simulink model "dragrace"  (R2021a)
settings: Solver=FixedStepAuto  StartTime=0.0  StopTime=t_final  FixedStep=t_step  RelTol=1e-3
values from neighbouring files (symbols this model uses):
  c_R = 0.015    [data_analysis.m]
  F_Reib = 0    [data_analysis.m]
  gamma = 0    [data_analysis.m]
  lambda = 1    [data_analysis.m]
  m = 2000    [data_analysis.m]
  M_Brems = 0    [data_analysis.m]
  MaxBremsmoment = 1000    [data_analysis.m]
  r = 33.55    [data_analysis.m]
  S_0 = 0    [data_analysis.m]
  v_0 = 0    [data_analysis.m]
  v_L = 0    [data_analysis.m]
settings Model: Creator=62958  LastModifiedBy=62958
settings SolverCC: AlgebraicLoopSolver=TrustRegion
settings DebuggingCC: SFMachineParentedDataDiag=warning
settings HardwareCC: ProdHWDeviceType=AMD->x86-64 (Windows64)

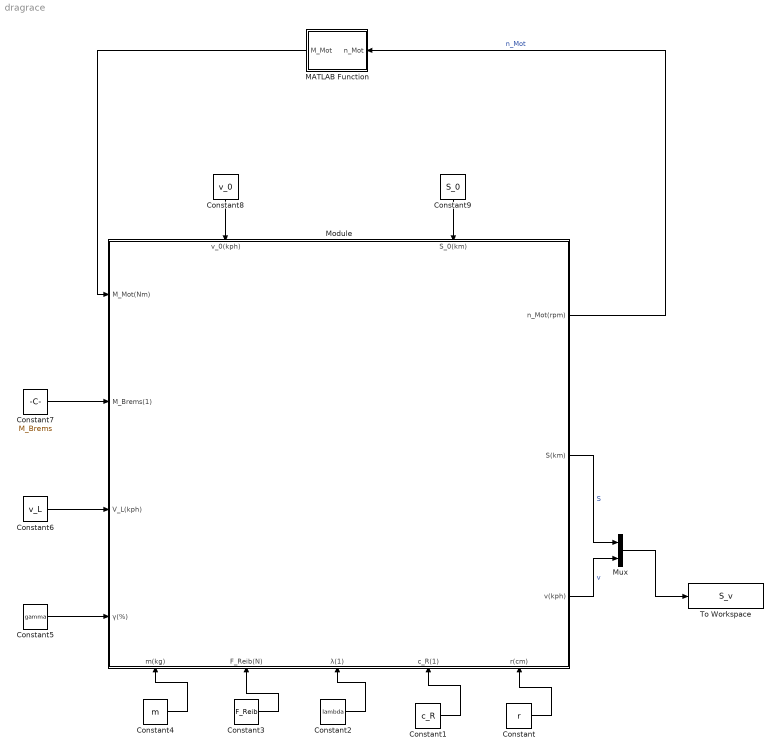
== system dragrace ==
  Constant : Constant  Value=r
  Constant1 : Constant  Value=c_R
  Constant2 : Constant  Value=lambda
  Constant3 : Constant  Value=F_Reib
  Constant4 : Constant  Value=m
  Constant5 : Constant  Value=gamma
  Constant6 : Constant  Value=v_L
  Constant7 : Constant  Value=M_Brems
  Constant8 : Constant  Value=v_0
  Constant9 : Constant  Value=S_0
  MATLAB Function : MATLAB Function  TreatAsAtomicUnit=on
  Module : Subsystem
      settings: PortSchema="{\"entries\":[{\"content\":{\"sides\":[{\"content\":{\"connectorIds\":[\"In1\",\"In2\",\"In3\",\"In4\"]},\"type\":\"ConnectorPlacement.EquallySpacedRectSide\",\"uuid\":\"ac678796-a959-4d6d-9319-846a0b7c832f\"},{\"content\":{\"connectorIds\":[\"Out1\",\"Out2\",\"Out3\"],\"side\":\"RIGHT\"},\"type\":\"ConnectorPlacement.EquallySpacedRectSide\",\"uuid\":\"19604558-b17b-4c8e-bdf8-e9ba0ab768c7\"},{\"content\":{\"connectorIds\":[\"In5\",\"In6\"],\"side\":\"TOP\"},\"type\":\"ConnectorPlacement.EquallySpacedRectSide\",\"uuid\":\"2ba52809-0b07-473f-b1d8-e379260c6f0c\"},{\"content\":{\"connectorIds\":[\"In7\",\"In8\",\"In9\",\"In10\",\"In11\"],\"side\":\"BOTTOM\"},\"type\":\"ConnectorPlacement.EquallySpacedRectSide\",\"uuid\":\"6dc63aca-051a-4fee-a312-85b6adf31509\"},{\"content\":{\"connectorIds\":[],\"side\":\"HIDDEN\"},\"type\":\"ConnectorPlacement.EquallySpacedRectSide\",\"uuid\":\"c73a095b-eeaa-49e3-925b-3fbd9f66e33c\"}]},\"type\":\"ConnectorPlacement.EquallySpacedConnector\",\"uuid\":\"c7629ab1-f4a5-46db-a10e-d6706fe7350a\"}],\"packageUris\":[\"http://schema.mathworks.com/mf0/Connector/R2020b\"],\"version\":\"1.0\"}"
  Mux : Mux  Inputs=2
  To Workspace : ToWorkspace  VariableName=S_v  SaveFormat=Timeseries  SampleTime=-1
  wires:
  MATLAB Function/1(M_Mot) -> Module/1(M_Mot(Nm))
  Module/1(n_Mot(rpm)) -> MATLAB Function/1(n_Mot)  "n_Mot"
  Module/3(v(kph)) -> Mux/2  "v"
  Constant/1 -> Module/11(r(cm))
  Constant1/1 -> Module/10(c_R(1))
  Constant2/1 -> Module/9(λ(1))
  Constant3/1 -> Module/8(F_Reib(N))
  Constant4/1 -> Module/7(m(kg))
  Constant5/1 -> Module/4(γ(%))
  Constant6/1 -> Module/3(V_L(kph))
  Constant7/1 -> Module/2(M_Brems(1))
  Constant8/1 -> Module/5(v_0(kph))
  Constant9/1 -> Module/6(S_0(km))
  Module/2(S(km)) -> Mux/1  "S"
  Mux/1 -> To Workspace/1

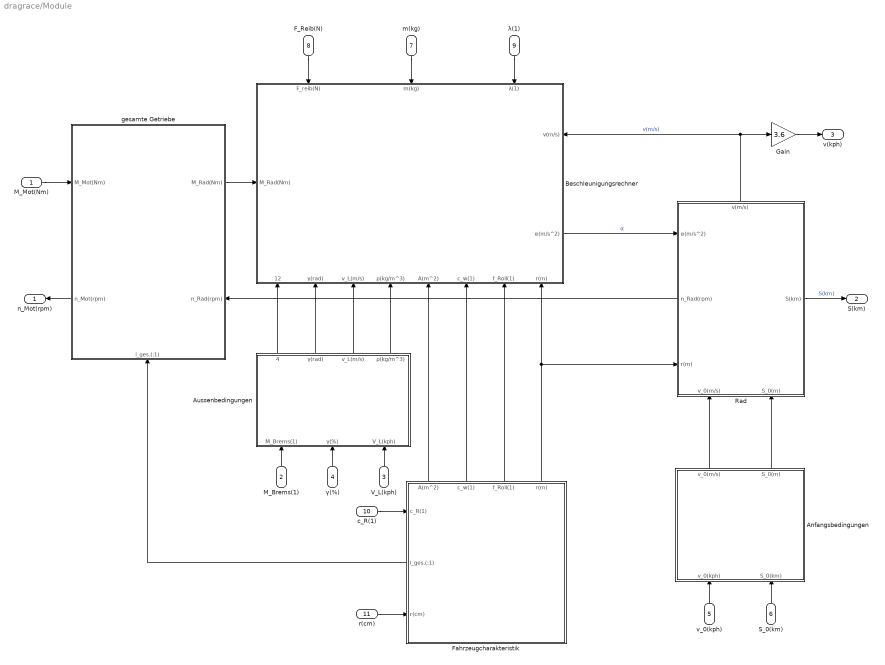
== system dragrace/Module ==
  M_Mot(Nm) : Inport
  M_Brems(1) : Inport  Port=2
  V_L(kph) : Inport  Port=3
  γ(%) : Inport  Port=4
  v_0(kph) : Inport  Port=5
  S_0(km) : Inport  Port=6
  m(kg) : Inport  Port=7
  F_Reib(N) : Inport  Port=8
  λ(1) : Inport  Port=9
  c_R(1) : Inport  Port=10
  r(cm) : Inport  Port=11
  Anfangsbedingungen : Subsystem
  Aussenbedingungen : Subsystem
      settings: PortSchema="{\"entries\":[{\"content\":{\"sides\":[{\"content\":{\"connectorIds\":[]},\"type\":\"ConnectorPlacement.EquallySpacedRectSide\",\"uuid\":\"b733fa8f-5d00-494c-b34f-88b15d5a1e12\"},{\"content\":{\"connectorIds\":[],\"side\":\"RIGHT\"},\"type\":\"ConnectorPlacement.EquallySpacedRectSide\",\"uuid\":\"0860ef04-b928-4d53-b793-a96484e4cbe0\"},{\"content\":{\"connectorIds\":[\"Out1\",\"Out2\",\"Out3\",\"Out4\"],\"side\":\"TOP\"},\"type\":\"ConnectorPlacement.EquallySpacedRectSide\",\"uuid\":\"090c1db3-6356-4eaa-9d0b-055902e2f27b\"},{\"content\":{\"connectorIds\":[\"In1\",\"In2\",\"In3\"],\"side\":\"BOTTOM\"},\"type\":\"ConnectorPlacement.EquallySpacedRectSide\",\"uuid\":\"59190b0a-2250-4f57-8c29-4644eef2c409\"},{\"content\":{\"connectorIds\":[],\"side\":\"HIDDEN\"},\"type\":\"ConnectorPlacement.EquallySpacedRectSide\",\"uuid\":\"ec20f46d-06e3-4d0a-9c7e-927ffb9f63c9\"}]},\"type\":\"ConnectorPlacement.EquallySpacedConnector\",\"uuid\":\"5c9482c8-38cc-4f92-88a5-86b3dbc9bf94\"}],\"packageUris\":[\"http://schema.mathworks.com/mf0/Connector/R2020b\"],\"version\":\"1.0\"}"
  Beschleunigungsrechner : Subsystem
      settings: PortSchema="{\"entries\":[{\"content\":{\"sides\":[{\"content\":{\"connectorIds\":[\"In1\",\"Out1\"]},\"type\":\"ConnectorPlacement.EquallySpacedRectSide\",\"uuid\":\"b733fa8f-5d00-494c-b34f-88b15d5a1e12\"},{\"content\":{\"connectorIds\":[\"In13\"],\"side\":\"RIGHT\"},\"type\":\"ConnectorPlacement.EquallySpacedRectSide\",\"uuid\":\"0860ef04-b928-4d53-b793-a96484e4cbe0\"},{\"content\":{\"connectorIds\":[\"In2\",\"In3\",\"In4\"],\"side\":\"TOP\"},\"type\":\"ConnectorPlacement.EquallySpacedRectSide\",\"uuid\":\"090c1db3-6356-4eaa-9d0b-055902e2f27b\"},{\"content\":{\"connectorIds\":[\"In5\",\"In6\",\"In7\",\"In8\",\"In9\",\"In10\",\"In11\",\"In12\"],\"side\":\"BOTTOM\"},\"type\":\"ConnectorPlacement.EquallySpacedRectSide\",\"uuid\":\"59190b0a-2250-4f57-8c29-4644eef2c409\"},{\"content\":{\"connectorIds\":[],\"side\":\"HIDDEN\"},\"type\":\"ConnectorPlacement.EquallySpacedRectSide\",\"uuid\":\"ec20f46d-06e3-4d0a-9c7e-927ffb9f63c9\"}]},\"type\":\"ConnectorPlacement.EquallySpacedConnector\",\"uuid\":\"5c9482c8-38cc-4f92-88a5-86b3dbc9bf94\"}],\"packageUris\":[\"http://schema.mathworks.com/mf0/Connector/R2020b\"],\"version\":\"1.0\"}"
  Fahrzeugcharakteristik : Subsystem
      settings: PortSchema="{\"entries\":[{\"content\":{\"sides\":[{\"content\":{\"connectorIds\":[\"In1\",\"Out5\",\"In2\"]},\"type\":\"ConnectorPlacement.EquallySpacedRectSide\",\"uuid\":\"425210de-c24d-4735-89d6-da620fee91ae\"},{\"content\":{\"connectorIds\":[],\"side\":\"RIGHT\"},\"type\":\"ConnectorPlacement.EquallySpacedRectSide\",\"uuid\":\"2aa95b8b-744b-4218-9974-9819eac83ec9\"},{\"content\":{\"connectorIds\":[\"Out1\",\"Out2\",\"Out3\",\"Out4\"],\"side\":\"TOP\"},\"type\":\"ConnectorPlacement.EquallySpacedRectSide\",\"uuid\":\"44fb0172-403e-4023-85b6-026c89d7dec6\"},{\"content\":{\"connectorIds\":[],\"side\":\"BOTTOM\"},\"type\":\"ConnectorPlacement.EquallySpacedRectSide\",\"uuid\":\"bc456c0b-389c-4a76-9795-db963bccb4d0\"},{\"content\":{\"connectorIds\":[],\"side\":\"HIDDEN\"},\"type\":\"ConnectorPlacement.EquallySpacedRectSide\",\"uuid\":\"03215e6b-5de7-4733-a8b0-f647922a7984\"}]},\"type\":\"ConnectorPlacement.EquallySpacedConnector\",\"uuid\":\"d1bd5eef-fe53-4c9e-be8a-2ad764aa59c2\"}],\"packageUris\":[\"http://schema.mathworks.com/mf0/Connector/R2020b\"],\"version\":\"1.0\"}"
  Gain : Gain  Gain=3.6
  Rad : Subsystem
      settings: PortSchema="{\"entries\":[{\"content\":{\"sides\":[{\"content\":{\"connectorIds\":[\"In1\",\"Out3\",\"In2\"]},\"type\":\"ConnectorPlacement.EquallySpacedRectSide\",\"uuid\":\"c3417092-dc7c-4039-9e9c-c2a6b9640efa\"},{\"content\":{\"connectorIds\":[\"Out1\"],\"side\":\"RIGHT\"},\"type\":\"ConnectorPlacement.EquallySpacedRectSide\",\"uuid\":\"749acbb4-c656-4eff-a125-532591d5cf60\"},{\"content\":{\"connectorIds\":[\"Out2\"],\"side\":\"TOP\"},\"type\":\"ConnectorPlacement.EquallySpacedRectSide\",\"uuid\":\"92c07f50-a812-457a-9ad7-17c408d902db\"},{\"content\":{\"connectorIds\":[\"In3\",\"In4\"],\"side\":\"BOTTOM\"},\"type\":\"ConnectorPlacement.EquallySpacedRectSide\",\"uuid\":\"b98cd1e8-b633-4d79-aeaf-c664ca03f589\"},{\"content\":{\"connectorIds\":[],\"side\":\"HIDDEN\"},\"type\":\"ConnectorPlacement.EquallySpacedRectSide\",\"uuid\":\"4099a9b5-4655-4782-9301-3d866c99b02b\"}]},\"type\":\"ConnectorPlacement.EquallySpacedConnector\",\"uuid\":\"1fc2dbdd-5020-4d82-be08-5c03d0ed68f0\"}],\"packageUris\":[\"http://schema.mathworks.com/mf0/Connector/R2020b\"],\"version\":\"1.0\"}"
  gesamte Getriebe : Subsystem
      settings: PortSchema="{\"entries\":[{\"content\":{\"sides\":[{\"content\":{\"connectorIds\":[\"In1\",\"Out2\"]},\"type\":\"ConnectorPlacement.EquallySpacedRectSide\",\"uuid\":\"b733fa8f-5d00-494c-b34f-88b15d5a1e12\"},{\"content\":{\"connectorIds\":[\"Out1\",\"In3\"],\"side\":\"RIGHT\"},\"type\":\"ConnectorPlacement.EquallySpacedRectSide\",\"uuid\":\"0860ef04-b928-4d53-b793-a96484e4cbe0\"},{\"content\":{\"connectorIds\":[],\"side\":\"TOP\"},\"type\":\"ConnectorPlacement.EquallySpacedRectSide\",\"uuid\":\"090c1db3-6356-4eaa-9d0b-055902e2f27b\"},{\"content\":{\"connectorIds\":[\"In2\"],\"side\":\"BOTTOM\"},\"type\":\"ConnectorPlacement.EquallySpacedRectSide\",\"uuid\":\"88222426-d39d-4ff1-9ccf-26b03ee0e8eb\"},{\"content\":{\"connectorIds\":[],\"side\":\"HIDDEN\"},\"type\":\"ConnectorPlacement.EquallySpacedRectSide\",\"uuid\":\"ec20f46d-06e3-4d0a-9c7e-927ffb9f63c9\"}]},\"type\":\"ConnectorPlacement.EquallySpacedConnector\",\"uuid\":\"5c9482c8-38cc-4f92-88a5-86b3dbc9bf94\"}],\"packageUris\":[\"http://schema.mathworks.com/mf0/Connector/R2020b\"],\"version\":\"1.0\"}"
  n_Mot(rpm) : Outport
  S(km) : Outport  Port=2
  v(kph) : Outport  Port=3
  wires:
  Fahrzeugcharakteristik/4(r(m)) -> Rad/2(r(m)), Beschleunigungsrechner/5(r(m))
  M_Mot(Nm)/1 -> gesamte Getriebe/1(M_Mot(Nm))
  Aussenbedingungen/2(v_L(m/s)) -> Beschleunigungsrechner/10(v_L(m/s))
  Rad/1(S(km)) -> S(km)/1  "S(km)"
  M_Brems(1)/1 -> Aussenbedingungen/3(M_Brems(1))
  gesamte Getriebe/2(n_Mot(rpm)) -> n_Mot(rpm)/1
  Aussenbedingungen/3(γ(rad)) -> Beschleunigungsrechner/11(γ(rad))
  Fahrzeugcharakteristik/5(i_ges.(:1)) -> gesamte Getriebe/2(i_ges.(:1))
  Anfangsbedingungen/1(v_0(m/s)) -> Rad/3(v_0(m/s))
  Aussenbedingungen/1(ρ(kg/m^3)) -> Beschleunigungsrechner/9(ρ(kg/m^3))
  gesamte Getriebe/1(M_Rad(Nm)) -> Beschleunigungsrechner/13(M_Rad(Nm))
  Fahrzeugcharakteristik/2(c_w(1)) -> Beschleunigungsrechner/7(c_w(1))
  Fahrzeugcharakteristik/1(A(m^2)) -> Beschleunigungsrechner/8(A(m^2))
  Anfangsbedingungen/2(S_0(m)) -> Rad/4(S_0(m))
  Fahrzeugcharakteristik/3(f_Roll(1)) -> Beschleunigungsrechner/6(f_Roll(1))
  Beschleunigungsrechner/1(α(m/s^2)) -> Rad/1(α(m/s^2))  "α"
  Rad/3(n_Rad(rpm)) -> gesamte Getriebe/3(n_Rad(rpm))
  Rad/2(v(m/s)) -> Gain/1, Beschleunigungsrechner/1(v(m/s))  "v(m/s)"
  γ(%)/1 -> Aussenbedingungen/2(γ(%))
  V_L(kph)/1 -> Aussenbedingungen/1(V_L(kph))
  F_Reib(N)/1 -> Beschleunigungsrechner/4(F_reib(N))
  c_R(1)/1 -> Fahrzeugcharakteristik/1(c_R(1))
  r(cm)/1 -> Fahrzeugcharakteristik/2(r(cm))
  v_0(kph)/1 -> Anfangsbedingungen/1(v_0(kph))
  S_0(km)/1 -> Anfangsbedingungen/2(S_0(km))
  m(kg)/1 -> Beschleunigungsrechner/3(m(kg))
  λ(1)/1 -> Beschleunigungsrechner/2(λ(1))
  Gain/1 -> v(kph)/1
  Aussenbedingungen/4(M_Brems(Nm)) -> Beschleunigungsrechner/12(M_Brems(Nm))

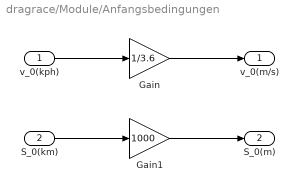
== system dragrace/Module/Anfangsbedingungen ==
  v_0(kph) : Inport
  S_0(km) : Inport  Port=2
  Gain : Gain  Gain=1/3.6
  Gain1 : Gain  Gain=1000
  v_0(m/s) : Outport
  S_0(m) : Outport  Port=2
  wires:
  Gain/1 -> v_0(m/s)/1
  v_0(kph)/1 -> Gain/1
  S_0(km)/1 -> Gain1/1
  Gain1/1 -> S_0(m)/1

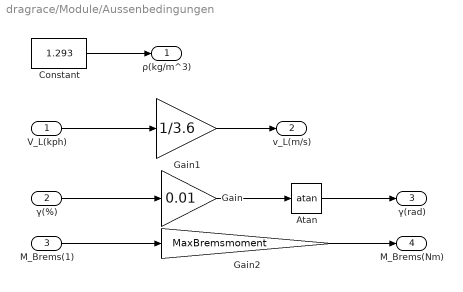
== system dragrace/Module/Aussenbedingungen ==
  V_L(kph) : Inport
  γ(%) : Inport  Port=2
  M_Brems(1) : Inport  Port=3
  Atan : Trigonometry  Operator=atan
  Constant : Constant  Value=1.293
  Gain : Gain  Gain=0.01
  Gain1 : Gain  Gain=1/3.6
  Gain2 : Gain  Gain=MaxBremsmoment
  ρ(kg/m^3) : Outport
  v_L(m/s) : Outport  Port=2
  γ(rad) : Outport  Port=3
  M_Brems(Nm) : Outport  Port=4
  wires:
  V_L(kph)/1 -> Gain1/1
  γ(%)/1 -> Gain/1
  Atan/1 -> γ(rad)/1
  Gain1/1 -> v_L(m/s)/1
  Gain/1 -> Atan/1
  Constant/1 -> ρ(kg/m^3)/1
  Gain2/1 -> M_Brems(Nm)/1
  M_Brems(1)/1 -> Gain2/1

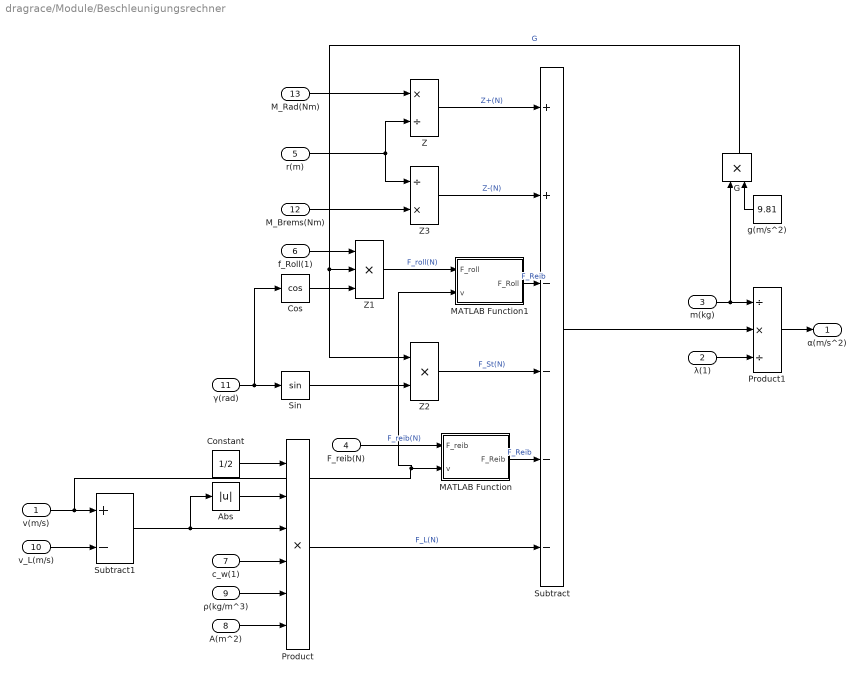
== system dragrace/Module/Beschleunigungsrechner ==
  v(m/s) : Inport
  λ(1) : Inport  Port=2
  m(kg) : Inport  Port=3
  F_reib(N) : Inport  Port=4
  r(m) : Inport  Port=5
  f_Roll(1) : Inport  Port=6
  c_w(1) : Inport  Port=7
  A(m^2) : Inport  Port=8
  ρ(kg/m^3) : Inport  Port=9
  v_L(m/s) : Inport  Port=10
  γ(rad) : Inport  Port=11
  M_Brems(Nm) : Inport  Port=12
  M_Rad(Nm) : Inport  Port=13
  Abs : Abs
  Constant : Constant  Value=1/2
  Cos : Trigonometry  Operator=cos
  G : Product
  MATLAB Function : MATLAB Function  TreatAsAtomicUnit=on
  MATLAB Function1 : MATLAB Function  TreatAsAtomicUnit=on
  Product : Product  Inputs=6
  Product1 : Product  Inputs=/*/
  Sin : Trigonometry
  Subtract : Sum  Inputs=++----
  Subtract1 : Sum  Inputs=+-
  Z : Product  Inputs=*/
  Z1 : Product  Inputs=***
  Z2 : Product  Inputs=**
  Z3 : Product  Inputs=/*
  g(m/s^2) : Constant  Value=9.81
  α(m/s^2) : Outport
  wires:
  M_Rad(Nm)/1 -> Z/1
  r(m)/1 -> Z3/1, Z/2
  Z/1 -> Subtract/1  "Z+(N)"
  Product1/1 -> α(m/s^2)/1
  Subtract/1 -> Product1/2
  m(kg)/1 -> G/1, Product1/1
  λ(1)/1 -> Product1/3
  g(m/s^2)/1 -> G/2
  G/1 -> Z2/1, Z1/2  "G"
  Z1/1 -> MATLAB Function1/1(F_roll)  "F_roll(N)"
  f_Roll(1)/1 -> Z1/1
  Z2/1 -> Subtract/4  "F_St(N)"
  M_Brems(Nm)/1 -> Z3/2
  Z3/1 -> Subtract/2  "Z-(N)"
  v_L(m/s)/1 -> Subtract1/2
  v(m/s)/1 -> MATLAB Function1/2(v), MATLAB Function/2(v), Subtract1/1
  Subtract1/1 -> Product/3, Abs/1
  Constant/1 -> Product/1
  Abs/1 -> Product/2
  c_w(1)/1 -> Product/4
  ρ(kg/m^3)/1 -> Product/5
  A(m^2)/1 -> Product/6
  Product/1 -> Subtract/6  "F_L(N)"
  F_reib(N)/1 -> MATLAB Function/1(F_reib)  "F_reib(N)"
  Sin/1 -> Z2/2
  γ(rad)/1 -> Sin/1, Cos/1
  Cos/1 -> Z1/3
  MATLAB Function/1(F_Reib) -> Subtract/5  "F_Reib"
  MATLAB Function1/1(F_Roll) -> Subtract/3  "F_Reib"

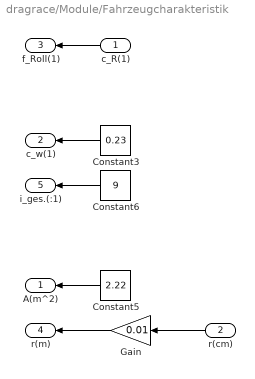
== system dragrace/Module/Fahrzeugcharakteristik ==
  c_R(1) : Inport
  r(cm) : Inport  Port=2
  Constant3 : Constant  Value=0.23
  Constant5 : Constant  Value=2.22
  Constant6 : Constant  Value=9
  Gain : Gain  Gain=0.01
  A(m^2) : Outport
  c_w(1) : Outport  Port=2
  f_Roll(1) : Outport  Port=3
  r(m) : Outport  Port=4
  i_ges.(:1) : Outport  Port=5
  wires:
  r(cm)/1 -> Gain/1
  Gain/1 -> r(m)/1
  c_R(1)/1 -> f_Roll(1)/1
  Constant6/1 -> i_ges.(:1)/1
  Constant5/1 -> A(m^2)/1
  Constant3/1 -> c_w(1)/1

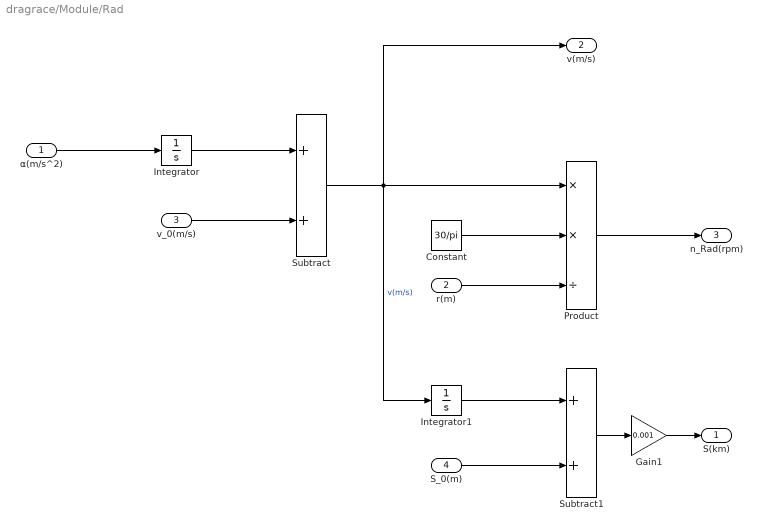
== system dragrace/Module/Rad ==
  α(m/s^2) : Inport
  r(m) : Inport  Port=2
  v_0(m/s) : Inport  Port=3
  S_0(m) : Inport  Port=4
  Constant : Constant  Value=30/pi
  Gain1 : Gain  Gain=0.001
  Integrator : Integrator
  Integrator1 : Integrator
  Product : Product  Inputs=**/
  Subtract : Sum
  Subtract1 : Sum
  S(km) : Outport
  v(m/s) : Outport  Port=2
  n_Rad(rpm) : Outport  Port=3
  wires:
  α(m/s^2)/1 -> Integrator/1
  Subtract/1 -> v(m/s)/1, Integrator1/1, Product/1  "v(m/s)"
  Integrator/1 -> Subtract/1
  v_0(m/s)/1 -> Subtract/2
  S_0(m)/1 -> Subtract1/2
  Integrator1/1 -> Subtract1/1
  Subtract1/1 -> Gain1/1
  Constant/1 -> Product/2
  r(m)/1 -> Product/3
  Product/1 -> n_Rad(rpm)/1
  Gain1/1 -> S(km)/1

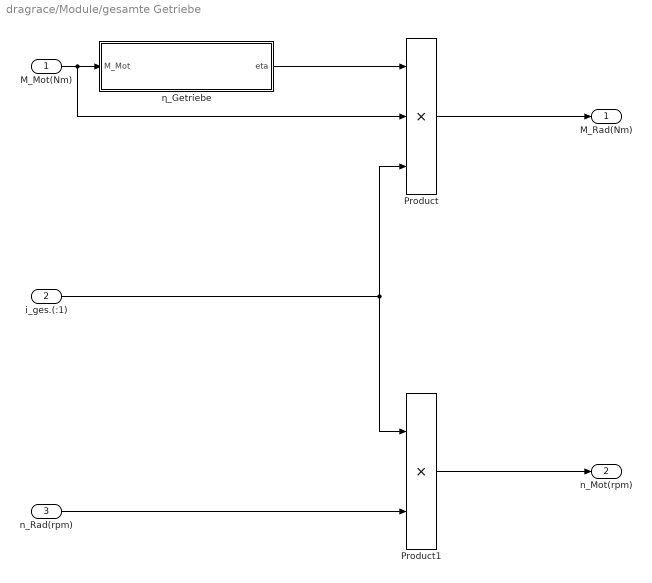
== system dragrace/Module/gesamte Getriebe ==
  M_Mot(Nm) : Inport
  i_ges.(:1) : Inport  Port=2
  n_Rad(rpm) : Inport  Port=3
  Product : Product  Inputs=***
  Product1 : Product
  η_Getriebe : MATLAB Function  TreatAsAtomicUnit=on
  M_Rad(Nm) : Outport
  n_Mot(rpm) : Outport  Port=2
  wires:
  Product/1 -> M_Rad(Nm)/1
  Product1/1 -> n_Mot(rpm)/1
  i_ges.(:1)/1 -> Product/3, Product1/1
  n_Rad(rpm)/1 -> Product1/2
  M_Mot(Nm)/1 -> η_Getriebe/1(M_Mot), Product/2
  η_Getriebe/1(eta) -> Product/1

== matlab function dragrace/Module/gesamte Getriebe/η_Getriebe ==
  data: M_Mot input; eta output
function eta = fcn(M_Mot)
eta_0=1;
if (M_Mot>0)%EM motorisch
    eta=1*eta_0;
elseif (M_Mot<0)%EM generatorisch
    eta=1/eta_0;
else%Leerlauf
    eta=1;
end

== matlab function dragrace/Module/Beschleunigungsrechner/MATLAB Function1 ==
  data: F_roll input; v input; F_Roll output
function F_Roll = fcn(F_roll,v)
if (v>0)
    F_Roll=F_roll;
elseif (v==0)
    F_Roll=0;
else
    F_Roll=-F_roll;
end

== matlab function dragrace/MATLAB Function ==
  data: n_Mot input; M_Mot output
function M_Mot = fcn(n_Mot)
n_tesla = [0 5000:1000:14000,20000,25000,25001];
M_tesla = [493,493,411,352.5,308.1,273.6,246.5,224.3,205.4,189.8,175.8,123.25,98.6,0];
M_Mot=interp1(n_tesla,M_tesla,n_Mot);

== matlab function dragrace/Module/Beschleunigungsrechner/MATLAB Function ==
  data: F_reib input; v input; F_Reib output
function F_Reib = fcn(F_reib,v)
if (v>0)
    F_Reib=F_reib;
elseif (v==0)
    F_Reib=0;
else
    F_Reib=-F_reib;
end
